simulink model "pid_ss_rl"  (R2022a)
settings: Solver=ode45  StartTime=0.0  StopTime=0.5  RelTol=1e-3  EnableMultiTasking=on
undefined symbols (not defined in the file or in its folder): DiscIntNeverNeededParam
libraries: simulink x1, rllib x1
settings Model: Creator=sneha  LastModifiedBy=archi
settings SolverCC: AlgebraicLoopSolver=TrustRegion
settings DataIOCC: LimitDataPoints=on  SaveFormat=Array
settings OptimizationCC: LifeSpan=inf
settings DebuggingCC: UnconnectedInputMsg=warning  UnconnectedOutputMsg=warning  UnconnectedLineMsg=warning  SFUnexpectedBacktrackingDiag=warning  SFNoUnconditionalDefaultTransitionDiag=warning  SFExecutionAtInitializationDiag=none  SFMachineParentedDataDiag=warning  ArithmeticOperatorsInVariantConditions=warning
settings HardwareCC: ProdBitPerPointer=32  ProdBitPerSizeT=32  ProdBitPerPtrDiffT=32  ProdLargestAtomicFloat=None  ProdIntDivRoundTo=Undefined  ProdEndianess=Unspecified  ProdWordSize=32  ProdHWDeviceType=32-bit Generic
settings ModelReferenceCC: PropagateSignalLabelsOutOfModel=off
settings SFSimCC: SimUseLocalCustomCode=off  CustomCodeUndefinedFunction=UseInterfaceOnly
settings RTWCC: RTWUseLocalCustomCode=off
settings CodeAppCC: StateflowObjectComments=on
settings GRTTargetCC: TargetLangStandard=C89/C90 (ANSI)
settings ConfigComp: CovMetricSettings=dw  CovSaveCumulativeToWorkspaceVar=on  CovSaveSingleToWorkspaceVar=on  CovExternalEMLEnable=off

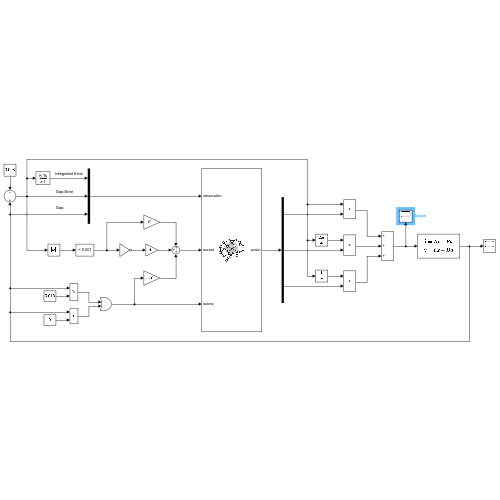
[thumbnail: Simulink's stored preview of the top-level diagram]
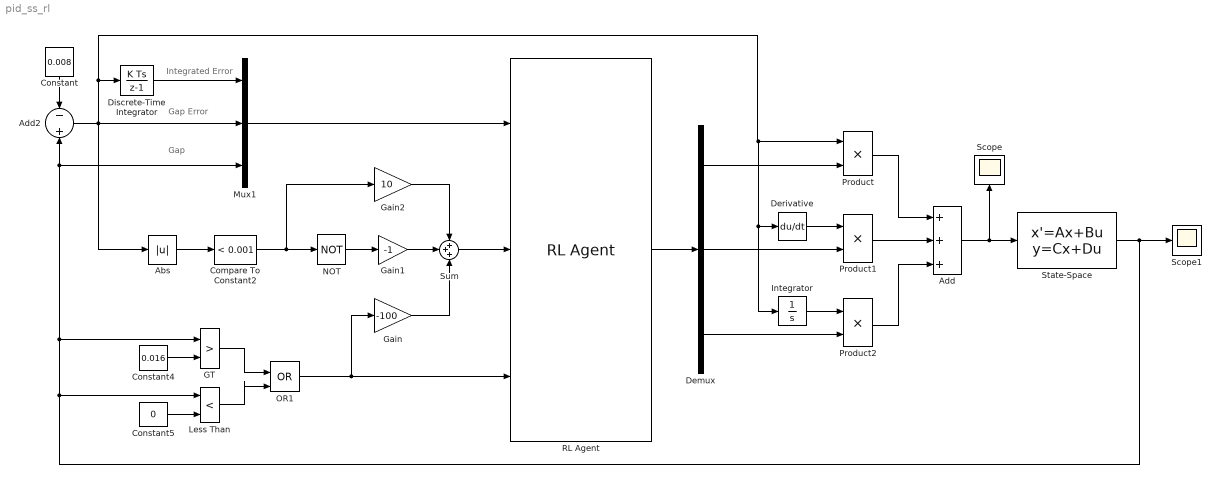
== system pid_ss_rl ==
  note: Gap
  note: Gap Error
  note: Integrated Error
  Abs : Abs  SaturateOnIntegerOverflow=off
  Add : Sum  Inputs=+++
  Add2 : Sum  Inputs=-|+
  Compare To Constant2 : simulink/Logic and Bit Operations/Compare To Constant  relop=<  const=0.001  OutDataTypeStr=boolean
  Constant : Constant  Value=0.008
  Constant4 : Constant  Value=0.016
  Constant5 : Constant  Value=0
  Demux : Demux  Outputs=3
  Derivative : Derivative
  Discrete-Time Integrator : DiscreteIntegrator  SampleTime=-1  ICPrevOutput=DiscIntNeverNeededParam  ICPrevScaledInput=DiscIntNeverNeededParam
  GT : RelationalOperator  Operator=>  OutDataTypeStr=boolean  RndMeth=Simplest  InputSameDT=off
  Gain : Gain  Gain=-100
  Gain1 : Gain  Gain=-1
  Gain2 : Gain  Gain=10
  Integrator : Integrator
  Less Than : RelationalOperator  Operator=<  OutDataTypeStr=boolean  RndMeth=Simplest  InputSameDT=off
  Mux1 : Mux  Inputs=3
  NOT : Logic  Operator=NOT  IconShape=distinctive  AllPortsSameDT=off  OutDataTypeStr=boolean
  OR1 : Logic  Operator=OR  IconShape=distinctive  AllPortsSameDT=off  OutDataTypeStr=boolean
  Product : Product
  Product1 : Product
  Product2 : Product
  RL Agent : rllib/RL Agent  Agent=agent1_Trained  ExternalActionAsInput=off  ProvideLastAction=off  ProvideCumRwd=off  TreatAsDirectFeedthrough=on  UseStrictObservationDataTypes=off
  Scope : Scope
  Scope1 : Scope
  State-Space : StateSpace  A=[0 1 0; 2450 0 -1.1558; 0 2119.7 -3.1438]  B=[0; 0; 2.6198]  C=[1 0 0]  D=[0]  InitialCondition=[0.004; 0; 0]
  Sum : Sum  Inputs=+++
  wires:
  Constant/1 -> Add2/1
  Mux1/1 -> RL Agent/1
  Constant4/1 -> GT/2
  State-Space/1 -> Add2/2, Mux1/3, GT/1, Less Than/1, Scope1/1
  Constant5/1 -> Less Than/2
  GT/1 -> OR1/1
  Less Than/1 -> OR1/2
  OR1/1 -> RL Agent/3, Gain/1
  Gain1/1 -> Sum/2
  Add2/1 -> Integrator/1, Derivative/1, Product/1, Discrete-Time Integrator/1, Mux1/2, Abs/1
  Gain2/1 -> Sum/1
  NOT/1 -> Gain1/1
  Compare To Constant2/1 -> Gain2/1, NOT/1
  Gain/1 -> Sum/3
  Abs/1 -> Compare To Constant2/1
  Sum/1 -> RL Agent/2
  Discrete-Time Integrator/1 -> Mux1/1
  RL Agent/1 -> Demux/1
  Demux/1 -> Product/2
  Demux/2 -> Product1/2
  Demux/3 -> Product2/2
  Derivative/1 -> Product1/1
  Integrator/1 -> Product2/1
  Product1/1 -> Add/2
  Product/1 -> Add/1
  Product2/1 -> Add/3
  Add/1 -> State-Space/1, Scope/1
